simulink model "Autopilot_q_running1"  (R2021a)
settings: Solver=ode4  StartTime=0.0  StopTime=168  FixedStep=0.01  RelTol=1e-3
undefined symbols (not defined in the file or in its folder): Aero_cofficients, Earth, Plane_state_store, Structural_data, Thrust_data_store, WGS84
libraries: pid_lib x12, aerolibactuator x5, aerolibfltsims x2, aerolibanim x1, simulink x1, aerolibtransform2 x1, shared6dof x1, sim3dlib x1, uavsim3dlib x1
(part 3 of 3)

== matlab function Autopilot_q_running1/Autopilot Quad mode/Autopilot ==
  data: p_dot_d input; q_dot_d input; r_dot_d input; acc_d input; Tzf1 output; Tzf2 output; Tzf3 output; Tzf4 output; Tzb5 output; Tzb6 output; Tzb7 output; Tzb8 output; Tx9 output; Tx10 output; delta_e output; delta_a output; delta_r output; Plane_state input; aero_data input; structure_data input; Thrust input
function [Tzf1,Tzf2,Tzf3,Tzf4,Tzb5,Tzb6,Tzb7,Tzb8,Tx9,Tx10,delta_e,delta_a,delta_r]= Autopilot(p_dot_d,q_dot_d,r_dot_d,acc_d,Plane_state, aero_data, structure_data, Thrust)

Tzf1=Thrust(1);
Tzf2=Thrust(2);
Tzf3=Thrust(3);
Tzf4=Thrust(4);

Tzb5=Thrust(5);
Tzb6=Thrust(6);
Tzb7=Thrust(7);
Tzb8=Thrust(8);
Tx9=Thrust(9);
Tx10=Thrust(10);
delta_e=Thrust(11);
delta_a=Thrust(12);
delta_r=Thrust(13);

a_X_d=acc_d(1);
a_Y_d=acc_d(2);
a_Z_d=acc_d(3);




mass=structure_data(1,1);c=structure_data(1,2);b=structure_data(1,3);s=structure_data(1,4);
Ix=structure_data(1,5);Iy=structure_data(1,6);Iz=structure_data(1,7);
Ixy=structure_data(1,8);Ixz=structure_data(1,9);Iyz=structure_data(1,10);
x1=structure_data(1,11);x2=structure_data(1,12);y1=structure_data(1,13);y2=structure_data(1,14);
y3=structure_data(1,15);y4=structure_data(1,16);y5=structure_data(1,17);y6=structure_data(1,18);
y7=structure_data(1,19);y8=structure_data(1,20);y9=structure_data(1,21);y10=structure_data(1,22);
z1=structure_data(1,23);mb=structure_data(1,24);

T_by_W=2.0;

c0=Ix*Iz-Ixz^2; 
c1=Ixz*(Ix-Iy+Iz)/c0;    
c2=(Iz*(Iz-Iy)+Ixz^2)/c0;                                              
c3=Iz/c0;
c4=Ixz/c0;
c5=(Iz-Ix)/c0;
c6=Ixz/Iy;
c7=((Ix-Iy)*Ix + Ixz^2)/c0;
c8=Ix/c0;
c3_inv=1/c3;
c8_inv=1/c8;

CLo =aero_data(1,1); CL_alpha=aero_data(1,2);CL_beta=aero_data(1,3); CL_delta_e=aero_data(1,4); CL_delta_a=aero_data(1,5); CL_delta_r=aero_data(1,6); CL_p=aero_data(1,7);CL_q=aero_data(1,8);CL_r=aero_data(1,9);

Cdo =aero_data(1,1); Cd_alpha=aero_data(1,2);Cd_beta=aero_data(1,3); Cd_delta_e=aero_data(1,4); Cd_delta_a=aero_data(1,5); Cd_delta_r=aero_data(1,6); Cd_p=aero_data(1,7);Cd_q=aero_data(1,8);Cd_r=aero_data(1,9);

CYo =aero_data(1,1); CY_alpha=aero_data(1,2);CY_beta=aero_data(1,3); CY_delta_e=aero_data(1,4); CY_delta_a=aero_data(1,5); CY_delta_r=aero_data(1,6); CY_p=aero_data(1,7);CY_q=aero_data(1,8);CY_r=aero_data(1,9);

Clo =aero_data(1,1); Cl_alpha=aero_data(1,2);Cl_beta=aero_data(1,3); Cl_delta_e=aero_data(1,4); Cl_delta_a=aero_data(1,5); Cl_delta_r=aero_data(1,6); Cl_p=aero_data(1,7);Cl_q=aero_data(1,8);Cl_r=aero_data(1,9);

Cmo =aero_data(1,1); Cm_alpha=aero_data(1,2);Cm_beta=aero_data(1,3); Cm_delta_e=aero_data(1,4); Cm_delta_a=aero_data(1,5); Cm_delta_r=aero_data(1,6); Cm_p=aero_data(1,7);Cm_q=aero_data(1,8);Cm_r=aero_data(1,9);

Cno =aero_data(1,1); Cn_alpha=aero_data(1,2);Cn_beta=aero_data(1,3); Cn_delta_e=aero_data(1,4); Cn_delta_a=aero_data(1,5); Cn_delta_r=aero_data(1,6); Cn_p=aero_data(1,7);Cn_q=aero_data(1,8);Cn_r=aero_data(1,9);

Cd_brake=0.0;brake=0.0;g=9.81;
b1=0.0007488;
d1=0.00002828;
b1_inv=1.0/b1;

u=Plane_state(1);
v=Plane_state(2);
w=Plane_state(3);
p=Plane_state(4);
q=Plane_state(5);
r=Plane_state(6);
phi=Plane_state(7);
theta=Plane_state(8);
psi=Plane_state(9);
X=Plane_state(10);
Y=Plane_state(11);
Z=Plane_state(12);




rho=1.225;
        Tzf=Tzf2+Tzf3;
        Tzb=Tzb6+Tzb7;
        Tx=Tx9+Tx10;


R_v_v1=[cos(psi) sin(psi) 0; -sin(psi) cos(psi) 0; 0 0 1];
R_v1_v2=[cos(theta) 0 -sin(theta) ;0 1 0; sin(theta) 0 cos(theta)];
R_v2_b=[1 0 0;0 cos(phi) sin(phi) ;0 -sin(phi) cos(phi)];
R_v_b=R_v2_b*R_v1_v2*R_v_v1;



V_v=R_v_b'*[ u;  v;  w];
V_X=V_v(1);
V_Y=V_v(2);
V_Z=V_v(3);
wn=0.0;
we=0.0;
wd=0.0;
ppp = R_v_b*[V_X-wn;V_Y-we;V_Z-wd];
u_r=ppp(1);
v_r=ppp(2);
w_r=ppp(3);

V=sqrt(u_r^2+v_r^2+w_r^2);



if (u_r^2+v_r^2+w_r^2)<=0.01 
    alpha=0;
else
    alpha=atan2( w_r, u_r);
end


if norm(u_r) < 10^-3  && norm(v_r) < 10^-3 && norm(w_r) < 10^-3
    beta=0;
else
    beta = asin(v_r/sqrt(u_r^2+v_r^2+w_r^2));
end



R_b_s=[cos(alpha) 0 sin(alpha) ;0 1 0; -sin(alpha) 0 cos(alpha)]; 
R_s_w=[cos(beta) sin(beta) 0; -sin(beta) cos(beta) 0; 0 0 1];
R_w_b=(R_b_s)'*(R_s_w)';


AA=R_v_b*[ a_X_d;  a_Y_d;  a_Z_d];

u_dot_d=AA(1);
v_dot_d=AA(2);
w_dot_d=AA(3);

mg_b = R_v_b*[0 ;0; mass*g];
D=0.5*rho*V*V*s*(Cdo+Cd_alpha*abs(alpha)+Cd_delta_e*abs(delta_e)+ Cd_brake*abs(brake)) ;
D_b=R_w_b*[-D;0;0];

if V<0.1
    CL = CLo + CL_alpha*alpha + CL_delta_e*delta_e ;
else
    CL = CLo + CL_alpha*alpha + CL_delta_e*delta_e  + CL_q*q*c/(2*V) ;
end
L=0.5*rho*V*V*s*(CL);
L_b = R_w_b*[0;0;-L];
if abs(V)<0.1
    CY=CYo + CY_delta_r*delta_r + CY_beta*beta;
else
    CY=CYo + CY_delta_r*delta_r + CY_beta*beta + CY_r*r*b/(2*V);
end
FY=0.5*rho*V*V*s*(CY);

l_aero=0.5*rho*V^2*s*b*( Clo + Cl_delta_a*delta_a +Cl_delta_r*delta_r +Cl_beta*beta )+0.5*rho*V*s*b*(Cl_p*p*b/2+Cl_r*r*b/2);
m_aero=0.5*rho*V^2*s*c*( Cmo + Cm_alpha*alpha + Cm_delta_e*delta_e)+0.5*rho*V*s*c*Cm_q*q*c/2;
n_aero=0.5*rho*V^2*s*b*( Cno + Cn_delta_a*delta_a +Cn_delta_r*delta_r +Cn_beta*beta )+0.5*rho*V*s*b*(Cn_r*r*b/2+ Cn_p*p*b/2);

    
	l=l_aero - Tzf2*y2*cos(mb) - Tzf3*y3*cos(mb)   - Tzb6*y6*cos(mb) - Tzb7*y7*cos(mb);
	m=m_aero + Tzf*x1*cos(mb) + Tzb*x2*cos(mb) + Tx9*z1 + d1*Tzf2*b1_inv*sin(mb) - d1*Tzf3*b1_inv*sin(mb) - d1*Tzb6*b1_inv*sin(mb) + d1*Tzb7*b1_inv*sin(mb) ;
%	n=n_aero - Tx9_real*y9  - d1*Tzf2_real/b1 + d1*Tzf3_real/b1 + d1*Tzb6_real/b1 - d1*Tzb7_real/b1 ; //optimization
	n=n_aero - Tx9*y9 - Tx10*y10 + (Tzf2*x1*sin(mb) - Tzf3*x1*sin(mb) +  Tzb6*x2*sin(mb) - Tzb7*x2*sin(mb)) - d1*Tzf2*b1_inv*cos(mb) + d1*Tzf3*b1_inv*cos(mb)  + d1*Tzb6*b1_inv*cos(mb)  - d1*Tzb7*b1_inv*cos(mb)  ;



	fx = Tx9 + Tx10 + D_b(1)+ mg_b(1)+L_b(1);
	%%%%%%%%%%%%%%%%%%%%%%%%%%%%%%%%%%%%%%%%%%%%%%%%%%%%%%%%%%%%%%%%%%%%%%%%%%%
	fy = (Tzf2*sin(mb) - Tzf3*sin(mb) + Tzb6*sin(mb) - Tzb7*sin(mb)) + D_b(2) + mg_b(2) + FY + L_b(2);
	%%%%%%%%%%%%%%%%%%%%%%%%%%%%%%%%%%%%%%%%%%%%%%%%%%%%%%%%%%%%%%%%%%%%%%%%%%%
	fz = -Tzf*cos(mb) - Tzb*cos(mb) + mg_b(3)+D_b(3)+L_b(3);

    
    
    tam=[-b1*y2,-b1*y3,-b1*y6,-b1*y7; b1*x1,b1*x1,b1*x2,b1*x2; -d1,d1,d1,-d1; -b1,-b1,-b1,-b1];
    tbm=zeros(4,1);
    tbm(1)=(((p_dot_d - c1*p*q + c2*(q*r) -c4*n)*c3_inv) - l_aero);%//(((p_dot_d - c1*p*q + c2*(q*r) -c4*n)/c3) - l_aero)*w1*3/8
		tbm(2)=(((q_dot_d - c5*p*r + c6*(p*p-r*r))*Iy) - m_aero);%//(((q_dot_d - c5*p*r + c6*(p*p-r*r))*Iy) - m_aero)*w1/2
		tbm(3)=(((r_dot_d - c7*p*q + c1*(q*r) -c4*l)*c8_inv) - n_aero);%//(((r_dot_d - c7*p*q + c1*(q*r) -c4*l)/c8) - n_aero)*w1/2
    tbm(4)=(mass*w_dot_d - mg_b(3) - D_b(3) -L_b(3));%//(mass*w_dot_d - mg_b(3) - D_b(3) -L_b(3))/2
    omega_velocity=inv(tam)*tbm;
    
    for i=1:4
    if omega_velocity(i)<0.0
        omega_velocity(i)=0.0;
    end
    end
    	omega_2=sqrt(omega_velocity(1));
		omega_3=sqrt(omega_velocity(2));
		omega_6=sqrt(omega_velocity(3));
		omega_7=sqrt(omega_velocity(4));
		
		
		Tzf2=b1*omega_2^2;
		
		Tzf3=b1*omega_3^2;
		
		Tzb6=b1*omega_6^2;
	
		Tzb7=b1*omega_7^2;

        Tzf=Tzf2+Tzf3;
        Tzb=Tzb6+Tzb7;
        Tx=Tx9+Tx10;
        
        Tzf1=0.0;
        Tzf4=0.0;
        Tzb5=0.0;
        Tzb8=0.0;
        Tx9=0.0;
        Tx10=0.0;
        delta_e=0.0;
        delta_a=0.0;
        delta_r=0.0;
        
if(Tzf > (T_by_W*mass*g)/2.0)
		
			Tzf=(T_by_W*mass*g)/2.0;
end
		if(Tzf<= 0.0)
		
			Tzf=0.0;
        end

		if(Tzf2<=0.0)
		
			Tzf2=0.0;
        end
		if(Tzf3<= 0.0)
		
			Tzf3=0.0;
        end

		if(Tzb> (T_by_W*mass*g)/2.0)
		
			Tzb=(T_by_W*mass*g)/2.0;
        end



		if(Tzb6<= 0.0)
		
			Tzb6=0.0;
        end
		if(Tzb7<=0.0)
		
			Tzb7=0.0;
        end

		if(Tzb<= 0.0)
		
			Tzb=0.0;
        end
        
		if(Tx< 0.0)
		
			Tx=0.0;
        end
        
		if(Tx9 < 0.0)
		
			Tx9=0.0;
        end


		if(Tx>60.0)
		
			Tx=60.0;
        end

		if((Tx9)>60.0)
		
			Tx9=60.0;
        end
        
	if(Tx10 < 0.0)
	
		Tx10=0.0;
    end

		if(Tzf2>(T_by_W*mass*g)/4.0)
		
			Tzf2 =(T_by_W*mass*g)/4.0;
        end
		if(Tzf3>=(T_by_W*mass*g)/4.0)
		
			Tzf3 =(T_by_W*mass*g)/4.0;
        end

		if(Tzb6>=(T_by_W*mass*g)/4.0)
		
			Tzb6 =(T_by_W*mass*g)/4.0;
        end
		if(Tzb7>=(T_by_W*mass*g)/4.0)
		
			Tzb7 =(T_by_W*mass*g)/4.0;
        end

end
